simulink model "modelling"  (R2024b)
settings: Solver=VariableStepAuto  StartTime=0.0  StopTime=10.0  RelTol=1e-3
InitFcn:
  | Init
  | Observer_and_complementary_filter
undefined symbols (not defined in the file): body, C, denH, denHw, DiscIntNeverNeededParam, drv, dspblkCoreblockFVToolHelper, Fv, g, gbox, gcbh, M11, M22, mot, ms22g, numH, numHw, sens, Ts, wheel
libraries: simulink_extras x4
settings Model: Creator=UTENTE041019  LastModifiedBy=lucag

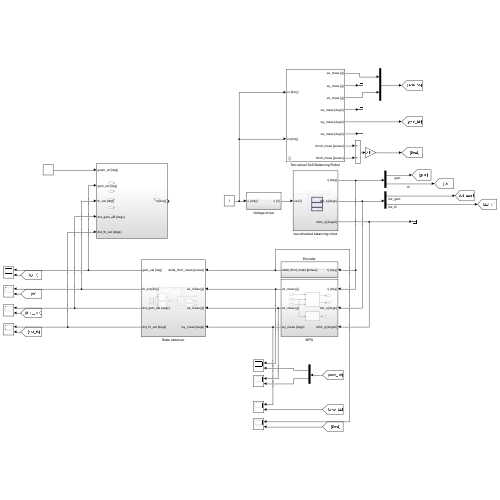
[thumbnail: Simulink's stored preview of the top-level diagram]
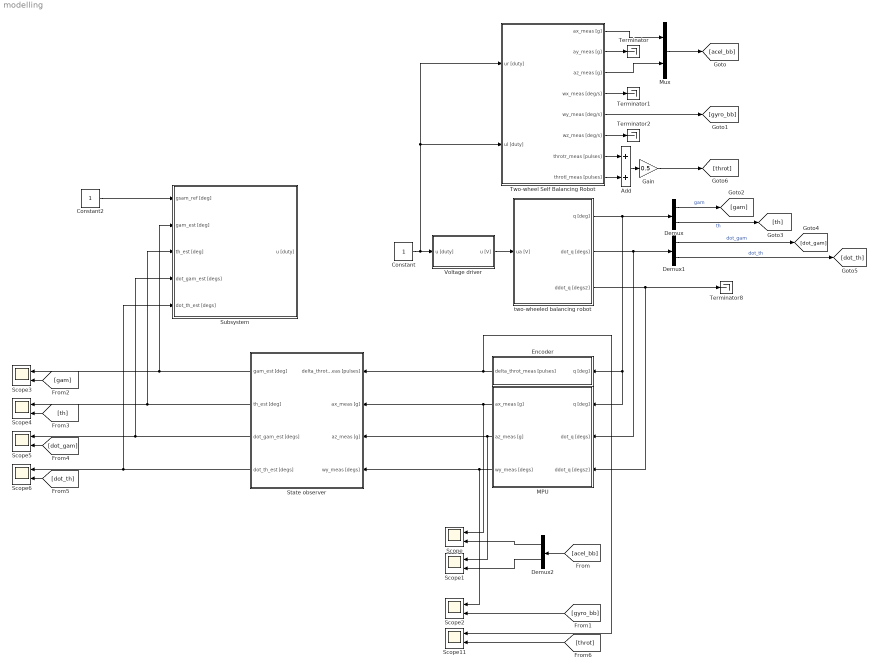
== system modelling ==
  Add : Sum
  Constant : Constant
  Constant2 : Constant
  Demux : Demux  Outputs=2
  Demux1 : Demux  Outputs=2
  Demux2 : Demux  Outputs=2
  Encoder : Subsystem
  Gain : Gain  Gain=0.5
  MPU : Subsystem
  Mux : Mux  Inputs=2
  Scope{,1..6,11} (8 alike) : Scope  NumInputPorts=2
  State observer : Subsystem
  Subsystem : Subsystem
  Terminator{,1..2,8} (4 alike) : Terminator
  "Two-wheel Self Balancing Robot " : Subsystem  mask(Balancing robot (longitudinal + lateral dynamics)){initState=[0, 0, 0, 0, 0, 0], Ts=0.01}
      mask prompts: initState "Initial state [gam(0), psi(0), th(0), dot_gam(0), dot_psi(0), dot_th(0)]'"; Ts "Sample time:"
      mask help:
      | Balancing robot dynamic model.
      | Includes both the longitudinal and lateral (yaw) dynamics.
      mask init:
      | %% General parameters and conversion gains
      | 
      | %   gravity acc [m/s^2]
      | g = 9.81;
      | 
      | %   conversion gains
      | rpm2rads = 2*pi/60;         %   [rpm]   -> [rad/s]
      | rads2rpm = 60/2/pi;         %   [rad/s] -> [rpm]
      | rpm2degs = 360/60;          %   [rpm]   -> [deg/s]
      | degs2rpm = 60/360;          %   [deg/s] -> [rpm]
      | deg2rad = pi/180;           %   [deg]   -> [rad]
      | rad2deg = 180/pi;           %   [rad]   -> [deg]
      | g2ms2 = g;                  %   [acc_g] -> [m/s^2]
      | ms22g = 1/g;                %   [m/s^2] -> [acc_g]
      | ozin2Nm = 0.706e-2;         %   [oz*inch] -> [N*m]
      | 
      | 
      | %%  Battery data
      | 
      | %   electrical data
      | batt.UN = 11.1;     %   nominal voltage
      | 
      | 
      | %%  H-bridge PWM voltage driver
      | 
      | drv.Vbus = batt.UN;                     %   H-bridge DC bus voltage  
      | drv.pwm.bits = 8;                       %   PWM resolution [bits]
      | drv.pwm.levels = 2^drv.pwm.bits;        %   PWM levels
      | drv.pwm.Fs = 490;                       %   PWM frequency
      | drv.dutymax = drv.pwm.levels-1;         %   max duty cycle code
      | drv.duty2V = drv.Vbus/drv.dutymax;      %   duty cycle code (0-255) to voltage
      | drv.V2duty = drv.dutymax/drv.Vbus;      %   voltage to duty cycle code (0-255)
      | 
      | 
      | %%  Gearbox data 
      | 
      | gbox.N = 30;            %   reduction ratio
      | 
      | 
      | %%  Sensors data - Hall-effect encoder
      | 
      | %   Hall-effect encoder
      | sens.enc.ppr = 16*4;    %   pulses per rotation at motor side (w/ quadrature decoding)
      | sens.enc.pulse2deg = 360/sens.enc.ppr;
      | sens.enc.pulse2rad = 2*pi/sens.enc.ppr;
      | sens.enc.deg2pulse = sens.enc.ppr/360;
      | sens.enc.rad2pulse = sens.enc.ppr/2/pi;
      | 
      | 
      | %%  Sensors data - MPU6050 (accelerometer + gyro)
      | 
      | %   center of mass (CoM) position
      | sens.mpu.xb = 0;
      | sens.mpu.yb = 0;
      | sens.mpu.zb = 13.5e-3;
      | 
      | %       MPU6050 embedded accelerometer specs
      | sens.mpu.acc.bits = 16;
      | sens.mpu.acc.fs_g = 16;                                                         %   full-scale in "g" units
      | sens.mpu.acc.fs = sens.mpu.acc.fs_g * g2ms2;                                    %   full-scale in [m/s^2] 
      | sens.mpu.acc.g2LSB = floor(2^(sens.mpu.acc.bits-1)/sens.mpu.acc.fs_g);          %   sensitivity [LSB/g]
      | sens.mpu.acc.ms22LSB = sens.mpu.acc.g2LSB * ms22g;                              %   sensitvity [LSB/(m/s^2)]
      | sens.mpu.acc.LSB2g = sens.mpu.acc.fs_g/2^(sens.mpu.acc.bits-1);                 %   output quantization step [g/LSB]
      | sens.mpu.acc.LSB2ms2 = sens.mpu.acc.LSB2g * g2ms2;                              %   output quantization step [ms2/LSB]
      | sens.mpu.acc.bw = 94;                                                           %   output low-pass filter bandwidth
      | sens.mpu.acc.noisestd = 400e-6*sqrt(100);                                       %   output noise std [g-rms]
      | sens.mpu.acc.noisevar = sens.mpu.acc.noisestd^2;                                %   output noise var [g^2]
      | 
      | %       MPU6050 embdedded gyroscope specs
      | sens.mpu.gyro.bits = 16;
      | sens.mpu.gyro.fs_degs = 250;                                                    %   full scale in [deg/s (dps)]
      | sens.mpu.gyro.fs = sens.mpu.gyro.fs_degs * deg2rad;                             %   full scale in [rad/s]
      | sens.mpu.gyro.degs2LSB = floor(2^(sens.mpu.gyro.bits-1)/sens.mpu.gyro.fs_degs);	%   sensitivity [LSB/degs]
      | sens.mpu.gyro.rads2LSB = sens.mpu.gyro.degs2LSB * rad2deg;                      %   sensitivity [LSB/rads] 
      | sens.mpu.gyro.LSB2degs = sens.mpu.gyro.fs_degs/2^(sens.mpu.gyro.bits-1);        %   output quantization step [degs/LSB]
      | sens.mpu.gyro.LSB2rads = sens.mpu.gyro.LSB2degs * deg2rad;                      %   output quantization step [rads/LSB]
      | sens.mpu.gyro.bw = 98;                                                          %   output low-pass filter bandwidth
      | sens.mpu.gyro.noisestd = 5e-3*sqrt(100);                                        %   output noise std [degs-rms]
      | sens.mpu.gyro.noisevar = sens.mpu.acc.noisestd ^2;                              %   output noise var [degs^2]
      mask Help:
      | Riccardo Antonello (antonello@dei.unipd.it)
      | 
      | May 19, 2020
      | 
      | Dept. of Information Engineering, University of Padova
  Voltage driver : Subsystem
  two-wheeled balancing robot : Subsystem
  wires:
  Voltage driver/1(u [V]) -> two-wheeled balancing robot/1(ua [V])
  two-wheeled balancing robot/1(q [deg]) -> MPU/1(q [deg]), Encoder/1(q [deg]), Demux/1
  two-wheeled balancing robot/2(dot_q [degs]) -> MPU/2(dot_q [degs]), Demux1/1
  two-wheeled balancing robot/3(ddot_q [degs2]) -> Terminator8/1, MPU/3(ddot_q [degs2])
  Constant/1 -> "Two-wheel Self Balancing Robot "/1(ur [duty]), "Two-wheel Self Balancing Robot "/2(ul [duty]), Voltage driver/1(u [duty])
  Demux/1 -> [gam]  "gam"
  Demux/2 -> [th]  "th"
  Demux1/2 -> [dot_th]  "dot_th"
  Demux1/1 -> [dot_gam]  "dot_gam"
  Encoder/1(delta_throt_meas [pulses]) -> Scope11/1, State observer/1(delta_throt_meas [pulses])
  MPU/1(ax_meas [g]) -> Scope/1, State observer/2(ax_meas [g])
  MPU/2(az_meas [g]) -> Scope1/1, State observer/3(az_meas [g])
  MPU/3(wy_meas [degs]) -> Scope2/1, State observer/4(wy_meas [degs])
  State observer/1(gam_est [deg]) -> Scope3/1, Subsystem/2(gam_est [deg])
  State observer/2(th_est [deg]) -> Scope4/1, Subsystem/3(th_est [deg])
  State observer/3(dot_gam_est [degs]) -> Subsystem/4(dot_gam_est [degs]), Scope5/1
  State observer/4(dot_th_est [degs]) -> Subsystem/5(dot_th_est [degs]), Scope6/1
  Constant2/1 -> Subsystem/1(gsam_ref [deg])
  [acel_bb] -> Demux2/1
  Demux2/1 -> Scope/2
  Demux2/2 -> Scope1/2
  [gyro_bb] -> Scope2/2
  [gam] -> Scope3/2
  [th] -> Scope4/2
  [dot_gam] -> Scope5/2
  [dot_th] -> Scope6/2
  "Two-wheel Self Balancing Robot "/2(ay_meas [g]) -> Terminator/1
  "Two-wheel Self Balancing Robot "/4(wx_meas [deg/s]) -> Terminator1/1
  "Two-wheel Self Balancing Robot "/6(wz_meas [deg/s]) -> Terminator2/1
  "Two-wheel Self Balancing Robot "/7(throtr_meas [pulses]) -> Add/1
  "Two-wheel Self Balancing Robot "/8(throtl_meas [pulses]) -> Add/2
  Add/1 -> Gain/1
  "Two-wheel Self Balancing Robot "/1(ax_meas [g]) -> Mux/1
  "Two-wheel Self Balancing Robot "/3(az_meas [g]) -> Mux/2
  Mux/1 -> [acel_bb]
  "Two-wheel Self Balancing Robot "/5(wy_meas [deg/s]) -> [gyro_bb]
  Gain/1 -> [throt]
  [throt] -> Scope11/2

== system modelling/Encoder ==
  q [deg] : Inport
  Gain : Gain  Gain=[1 -1]  Multiplication=Matrix(K*u)
  Gain1 : Gain  Gain=gbox.N
  Gain2 : Gain  Gain=sens.enc.deg2pulse
  Quantizer : Quantizer  QuantizationInterval=sens.enc.pulse2deg
  Zero-Order Hold : ZeroOrderHold  SampleTime=Ts
  delta_throt_meas [pulses] : Outport
  wires:
  Quantizer/1 -> Gain2/1
  Gain1/1 -> Zero-Order Hold/1
  Zero-Order Hold/1 -> Quantizer/1
  Gain/1 -> Gain1/1
  q [deg]/1 -> Gain/1
  Gain2/1 -> delta_throt_meas [pulses]/1

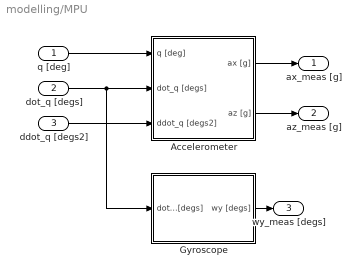
== system modelling/MPU ==
  q [deg] : Inport
  dot_q [degs] : Inport  Port=2
  ddot_q [degs2] : Inport  Port=3
  Accelerometer : Subsystem
  Gyroscope : Subsystem
  ax_meas [g] : Outport
  az_meas [g] : Outport  Port=2
  wy_meas [degs] : Outport  Port=3
  wires:
  dot_q [degs]/1 -> Gyroscope/1(dot_q [degs]), Accelerometer/2(dot_q [degs])
  ddot_q [degs2]/1 -> Accelerometer/3(ddot_q [degs2])
  Accelerometer/2(az [g]) -> az_meas [g]/1
  Accelerometer/1(ax [g]) -> ax_meas [g]/1
  Gyroscope/1(wy [degs]) -> wy_meas [degs]/1
  q [deg]/1 -> Accelerometer/1(q [deg])

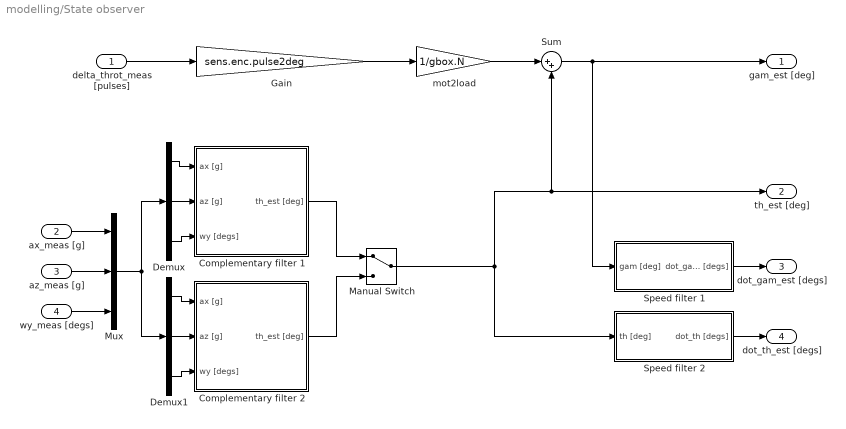
== system modelling/State observer ==
  delta_throt_meas [pulses] : Inport
  ax_meas [g] : Inport  Port=2
  az_meas [g] : Inport  Port=3
  wy_meas [degs] : Inport  Port=4
  Complementary filter 1 : Subsystem
  Complementary filter 2 : Subsystem
  Demux : Demux  Outputs=3
  Demux1 : Demux  Outputs=3
  Gain : Gain  Gain=sens.enc.pulse2deg
  Manual Switch : ManualSwitch
  Mux : Mux  Inputs=3
  Speed filter 1 : Subsystem
  Speed filter 2 : Subsystem
  Sum : Sum  Inputs=|++
  mot2load : Gain  Gain=1/gbox.N
  gam_est [deg] : Outport
  th_est [deg] : Outport  Port=2
  dot_gam_est [degs] : Outport  Port=3
  dot_th_est [degs] : Outport  Port=4
  wires:
  delta_throt_meas [pulses]/1 -> Gain/1
  Gain/1 -> mot2load/1
  mot2load/1 -> Sum/1
  Sum/1 -> Speed filter 1/1(gam [deg]), gam_est [deg]/1
  Speed filter 1/1(dot_gam [degs]) -> dot_gam_est [degs]/1
  Speed filter 2/1(dot_th [degs]) -> dot_th_est [degs]/1
  ax_meas [g]/1 -> Mux/1
  az_meas [g]/1 -> Mux/2
  wy_meas [degs]/1 -> Mux/3
  Demux/1 -> Complementary filter 1/1(ax [g])
  Demux/3 -> Complementary filter 1/3(wy [degs])
  Demux/2 -> Complementary filter 1/2(az [g])
  Demux1/2 -> Complementary filter 2/2(az [g])
  Demux1/1 -> Complementary filter 2/1(ax [g])
  Demux1/3 -> Complementary filter 2/3(wy [degs])
  Mux/1 -> Demux/1, Demux1/1
  Complementary filter 1/1(th_est [deg]) -> Manual Switch/1
  Complementary filter 2/1(th_est [deg]) -> Manual Switch/2
  Manual Switch/1 -> Sum/2, th_est [deg]/1, Speed filter 2/1(th [deg])

== system modelling/Subsystem ==
  gsam_ref [deg] : Inport
  gam_est [deg] : Inport  Port=2
  th_est [deg] : Inport  Port=3
  dot_gam_est [degs] : Inport  Port=4
  dot_th_est [degs] : Inport  Port=5
  u [duty] : Outport

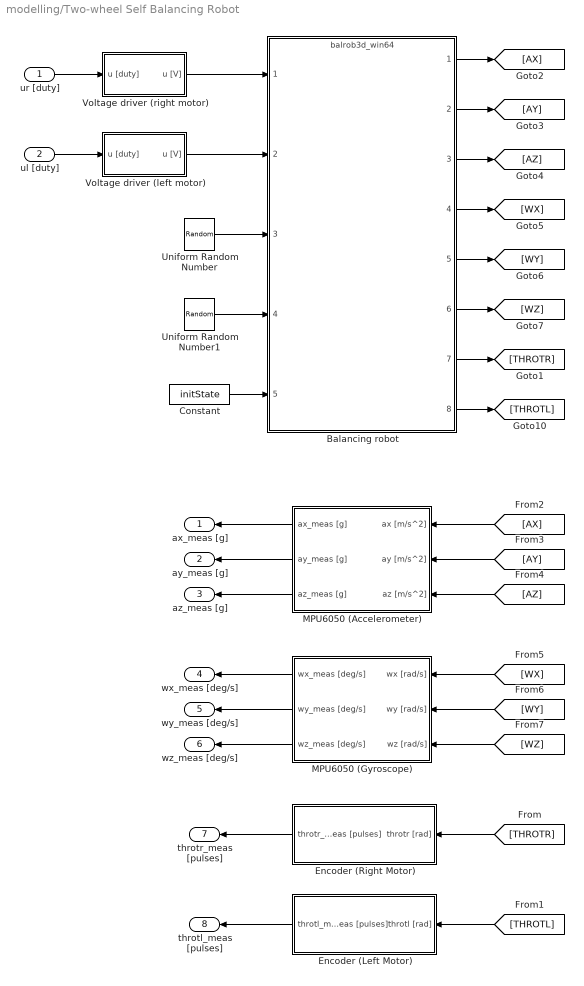
== system modelling/Two-wheel Self Balancing Robot  ==
  ur [duty] : Inport
  ul [duty] : Inport  Port=2
  Balancing robot : ModelReference  ModelNameDialog=balrob3d_win64.slxp  ModelReferenceVersion=1.741  CopyOfModelProtected=on
  Constant : Constant  Value=initState
  Encoder (Left Motor) : Subsystem
  Encoder (Right Motor) : Subsystem
  MPU6050 (Accelerometer) : Subsystem
  MPU6050 (Gyroscope) : Subsystem
  Uniform Random Number : UniformRandomNumber  Minimum=0.7  Maximum=1.3  SampleTime=1
  Uniform Random Number1 : UniformRandomNumber  Minimum=0.7  Maximum=1.3  Seed=10  SampleTime=1
  Voltage driver (left motor) : Subsystem
  Voltage driver (right motor) : Subsystem
  ax_meas [g] : Outport
  ay_meas [g] : Outport  Port=2
  az_meas [g] : Outport  Port=3
  wx_meas [deg/s] : Outport  Port=4
  wy_meas [deg/s] : Outport  Port=5
  wz_meas [deg/s] : Outport  Port=6
  throtr_meas [pulses] : Outport  Port=7
  throtl_meas [pulses] : Outport  Port=8
  wires:
  ur [duty]/1 -> Voltage driver (right motor)/1(u [duty])
  [WX] -> MPU6050 (Gyroscope)/1(wx [rad/s])
  Balancing robot/2 -> [AY]
  Balancing robot/4 -> [WX]
  Balancing robot/8 -> [THROTL]
  Balancing robot/1 -> [AX]
  [THROTL] -> Encoder (Left Motor)/1(throtl [rad])
  Balancing robot/6 -> [WZ]
  Balancing robot/7 -> [THROTR]
  Balancing robot/5 -> [WY]
  [AX] -> MPU6050 (Accelerometer)/1(ax [m/s^2])
  [WY] -> MPU6050 (Gyroscope)/2(wy [rad/s])
  Balancing robot/3 -> [AZ]
  [WZ] -> MPU6050 (Gyroscope)/3(wz [rad/s])
  [AZ] -> MPU6050 (Accelerometer)/3(az [m/s^2])
  [THROTR] -> Encoder (Right Motor)/1(throtr [rad])
  ul [duty]/1 -> Voltage driver (left motor)/1(u [duty])
  [AY] -> MPU6050 (Accelerometer)/2(ay [m/s^2])
  MPU6050 (Accelerometer)/1(ax_meas [g]) -> ax_meas [g]/1
  MPU6050 (Accelerometer)/2(ay_meas [g]) -> ay_meas [g]/1
  MPU6050 (Accelerometer)/3(az_meas [g]) -> az_meas [g]/1
  MPU6050 (Gyroscope)/1(wx_meas [deg/s]) -> wx_meas [deg/s]/1
  MPU6050 (Gyroscope)/2(wy_meas [deg/s]) -> wy_meas [deg/s]/1
  MPU6050 (Gyroscope)/3(wz_meas [deg/s]) -> wz_meas [deg/s]/1
  Encoder (Right Motor)/1(throtr_meas [pulses]) -> throtr_meas [pulses]/1
  Encoder (Left Motor)/1(throtl_meas [pulses]) -> throtl_meas [pulses]/1
  Voltage driver (right motor)/1(u [V]) -> Balancing robot/1
  Voltage driver (left motor)/1(u [V]) -> Balancing robot/2
  Uniform Random Number/1 -> Balancing robot/3
  Uniform Random Number1/1 -> Balancing robot/4
  Constant/1 -> Balancing robot/5

== system modelling/Voltage driver ==
  u [duty] : Inport
  " " : Gain  Gain=drv.duty2V
  Rounding Function : Rounding  Operator=fix
  Saturation : Saturate  UpperLimit=drv.dutymax  LowerLimit=-drv.dutymax
  Saturation1 : Saturate  UpperLimit=drv.Vbus  LowerLimit=-drv.Vbus
  Zero-Order Hold : ZeroOrderHold  SampleTime=Ts
  u [V] : Outport
  wires:
  Rounding Function/1 -> " "/1
  " "/1 -> Saturation1/1
  Saturation1/1 -> Zero-Order Hold/1
  u [duty]/1 -> Saturation/1
  Saturation/1 -> Rounding Function/1
  Zero-Order Hold/1 -> u [V]/1

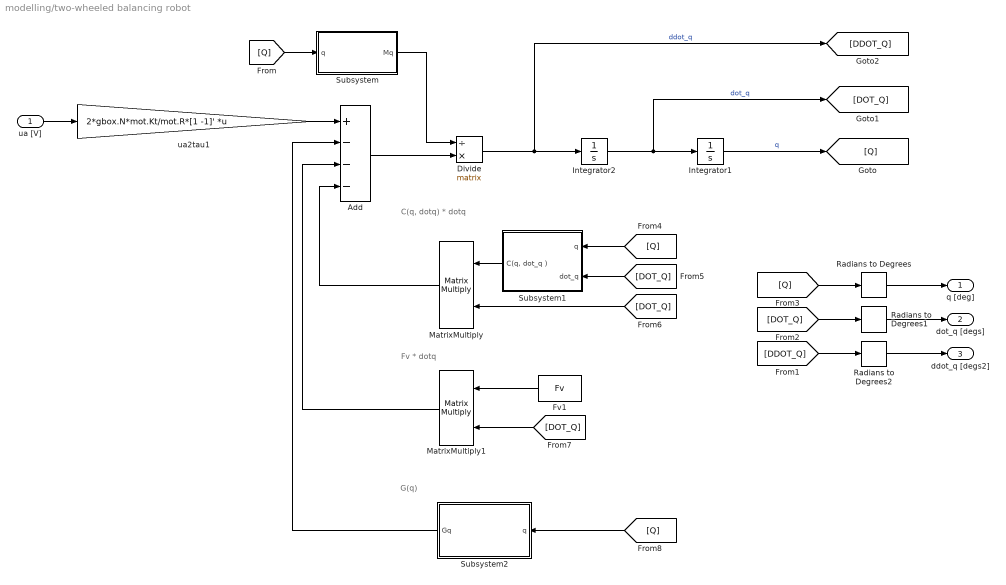
== system modelling/two-wheeled balancing robot ==
  note: G(q)
  note: Fv * dotq
  note: C(q, dotq) * dotq
  ua [V] : Inport
  Add : Sum  Inputs=+---
  Divide : Product  Inputs=/*  Multiplication=Matrix(*)
  Fv1 : Constant  Value=Fv
  Integrator1 : Integrator  InitialCondition=[0 0]'
  Integrator2 : Integrator  InitialCondition=[0 0]'
  MatrixMultiply : Product  Multiplication=Matrix(*)
  MatrixMultiply1 : Product  Multiplication=Matrix(*)
  Radians to Degrees : simulink_extras/Transformations/Radians to Degrees
  Radians to Degrees1 : simulink_extras/Transformations/Radians to Degrees
  Radians to Degrees2 : simulink_extras/Transformations/Radians to Degrees
  Subsystem : Subsystem
  Subsystem1 : Subsystem
  Subsystem2 : Subsystem
  ua2tau1 : Gain  Gain=2*gbox.N*mot.Kt/mot.R*[1 -1]'  Multiplication=Matrix(K*u)
  q [deg] : Outport
  dot_q [degs] : Outport  Port=2
  ddot_q [degs2] : Outport  Port=3
  wires:
  Subsystem1/1("C(q, dot_q )") -> MatrixMultiply/1
  Integrator2/1 -> [DOT_Q], Integrator1/1  "dot_q"
  Add/1 -> Divide/2
  [DOT_Q] -> Radians to Degrees1/1
  Divide/1 -> Integrator2/1, [DDOT_Q]  "ddot_q"
  Integrator1/1 -> [Q]  "q"
  ua2tau1/1 -> Add/1
  Radians to Degrees/1 -> q [deg]/1
  ua [V]/1 -> ua2tau1/1
  [Q] -> Subsystem1/1(q)
  Radians to Degrees1/1 -> dot_q [degs]/1
  Radians to Degrees2/1 -> ddot_q [degs2]/1
  [Q] -> Radians to Degrees/1
  [DDOT_Q] -> Radians to Degrees2/1
  MatrixMultiply/1 -> Add/4
  MatrixMultiply1/1 -> Add/3
  [DOT_Q] -> MatrixMultiply/2
  Subsystem2/1(Gq) -> Add/2
  [DOT_Q] -> MatrixMultiply1/2
  [Q] -> Subsystem/1(q)
  [DOT_Q] -> Subsystem1/2(dot_q)
  Subsystem/1(Mq) -> Divide/1
  [Q] -> Subsystem2/1(q)
  Fv1/1 -> MatrixMultiply1/1

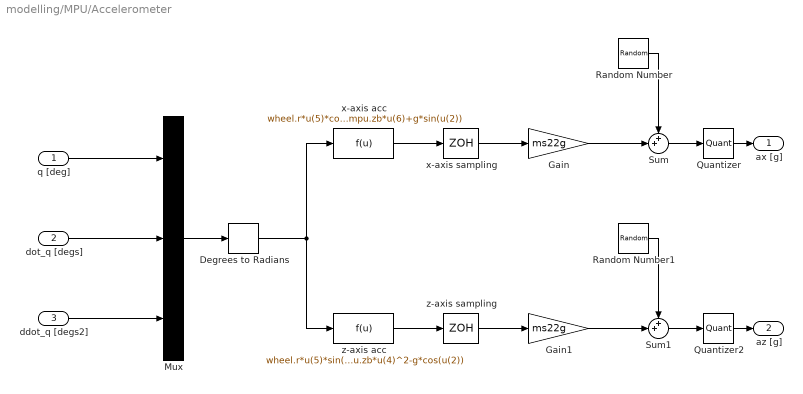
== system modelling/MPU/Accelerometer ==
  q [deg] : Inport
  dot_q [degs] : Inport  Port=2
  ddot_q [degs2] : Inport  Port=3
  Degrees to Radians : simulink_extras/Transformations/Degrees to Radians
  Gain : Gain  Gain=ms22g
  Gain1 : Gain  Gain=ms22g
  Mux : Mux  Inputs=3
  Quantizer : Quantizer  QuantizationInterval=sens.mpu.acc.LSB2g
  Quantizer2 : Quantizer  QuantizationInterval=sens.mpu.acc.LSB2g
  Random Number : RandomNumber  Variance=sens.mpu.acc.noisevar  SampleTime=Ts
  Random Number1 : RandomNumber  Variance=sens.mpu.acc.noisevar  SampleTime=Ts
  Sum : Sum  Inputs=++|
  Sum1 : Sum  Inputs=++|
  x-axis acc : Fcn  Expr=wheel.r*u(5)*cos(u(2))+sens.mpu.zb*u(6)+g*sin(u(2))
  x-axis sampling : ZeroOrderHold  SampleTime=Ts
  z-axis acc : Fcn  Expr=wheel.r*u(5)*sin(u(2))-sens.mpu.zb*u(4)^2-g*cos(u(2))
  z-axis sampling : ZeroOrderHold  SampleTime=Ts
  ax [g] : Outport
  az [g] : Outport  Port=2
  wires:
  Quantizer2/1 -> az [g]/1
  Gain/1 -> Sum/2
  Sum/1 -> Quantizer/1
  Random Number1/1 -> Sum1/1
  x-axis acc/1 -> x-axis sampling/1
  ddot_q [degs2]/1 -> Mux/3
  z-axis sampling/1 -> Gain1/1
  Sum1/1 -> Quantizer2/1
  Gain1/1 -> Sum1/2
  z-axis acc/1 -> z-axis sampling/1
  x-axis sampling/1 -> Gain/1
  Mux/1 -> Degrees to Radians/1
  dot_q [degs]/1 -> Mux/2
  Random Number/1 -> Sum/1
  Quantizer/1 -> ax [g]/1
  q [deg]/1 -> Mux/1
  Degrees to Radians/1 -> z-axis acc/1, x-axis acc/1

== system modelling/MPU/Gyroscope ==
  dot_q [degs] : Inport
  Quantizer1 : Quantizer  QuantizationInterval=sens.mpu.gyro.LSB2degs
  Random Number2 : RandomNumber  Variance=sens.mpu.gyro.noisevar  SampleTime=Ts
  Selector : Gain  Gain=[0 1]  Multiplication=Matrix(K*u)
  Sum2 : Sum  Inputs=++|
  Y-axis sampling : ZeroOrderHold  SampleTime=Ts
  wy [degs] : Outport
  wires:
  Selector/1 -> Y-axis sampling/1
  Sum2/1 -> Quantizer1/1
  Random Number2/1 -> Sum2/1
  Y-axis sampling/1 -> Sum2/2
  Quantizer1/1 -> wy [degs]/1
  dot_q [degs]/1 -> Selector/1

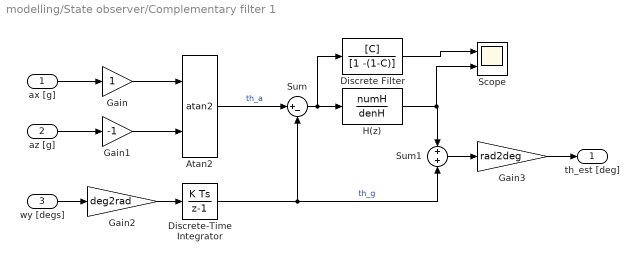
== system modelling/State observer/Complementary filter 1 ==
  ax [g] : Inport
  az [g] : Inport  Port=2
  wy [degs] : Inport  Port=3
  Atan2 : Trigonometry  Operator=atan2
  Discrete Filter : DiscreteFilter  LoadFcn=dspblkCoreblockFVToolHelper(gcbh,'load');  Numerator=[C]  Denominator=[1 -(1-C)]
      settings: CopyFcn=dspblkCoreblockFVToolHelper(gcbh,'copy');  DeleteFcn=dspblkCoreblockFVToolHelper(gcbh,'close');  ModelCloseFcn=dspblkCoreblockFVToolHelper(gcbh,'close');  PreSaveFcn=dspblkCoreblockFVToolHelper(gcbh,'presave');  PostSaveFcn=dspblkCoreblockFVToolHelper(gcbh,'postsave');  CloseFcn=dspblkCoreblockFVToolHelper(gcbh,'close');
  Discrete-Time Integrator : DiscreteIntegrator  SampleTime=Ts  ICPrevOutput=DiscIntNeverNeededParam  ICPrevScaledInput=DiscIntNeverNeededParam
  Gain : Gain
  Gain1 : Gain  Gain=-1
  Gain2 : Gain  Gain=deg2rad
  Gain3 : Gain  Gain=rad2deg
  H(z) : DiscreteTransferFcn  Numerator=numH  Denominator=denH
  Scope : Scope  NumInputPorts=2
  Sum : Sum  Inputs=|+-
  Sum1 : Sum  Inputs=+|+
  th_est [deg] : Outport
  wires:
  ax [g]/1 -> Gain/1
  az [g]/1 -> Gain1/1
  Gain/1 -> Atan2/1
  Gain1/1 -> Atan2/2
  Atan2/1 -> Sum/1  "th_a"
  wy [degs]/1 -> Gain2/1
  Gain2/1 -> Discrete-Time Integrator/1
  Discrete-Time Integrator/1 -> Sum1/2, Sum/2  "th_g"
  Sum/1 -> Discrete Filter/1, H(z)/1
  H(z)/1 -> Scope/2, Sum1/1
  Sum1/1 -> Gain3/1
  Gain3/1 -> th_est [deg]/1
  Discrete Filter/1 -> Scope/1

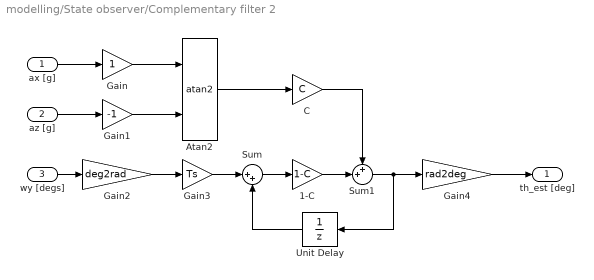
== system modelling/State observer/Complementary filter 2 ==
  ax [g] : Inport
  az [g] : Inport  Port=2
  wy [degs] : Inport  Port=3
  1-C : Gain  Gain=1-C
  Atan2 : Trigonometry  Operator=atan2
  C : Gain  Gain=C
  Gain : Gain
  Gain1 : Gain  Gain=-1
  Gain2 : Gain  Gain=deg2rad
  Gain3 : Gain  Gain=Ts
  Gain4 : Gain  Gain=rad2deg
  Sum : Sum  Inputs=|++
  Sum1 : Sum  Inputs=++|
  Unit Delay : UnitDelay  SampleTime=-1  HasFrameUpgradeWarning=on
  th_est [deg] : Outport
  wires:
  Gain/1 -> Atan2/1
  az [g]/1 -> Gain1/1
  Gain1/1 -> Atan2/2
  ax [g]/1 -> Gain/1
  Atan2/1 -> C/1
  wy [degs]/1 -> Gain2/1
  Gain2/1 -> Gain3/1
  Gain3/1 -> Sum/1
  Sum/1 -> 1-C/1
  C/1 -> Sum1/1
  1-C/1 -> Sum1/2
  Sum1/1 -> Unit Delay/1, Gain4/1
  Unit Delay/1 -> Sum/2
  Gain4/1 -> th_est [deg]/1

== system modelling/State observer/Speed filter 1 ==
  gam [deg] : Inport
  Discrete Transfer Fcn : DiscreteTransferFcn  Numerator=numHw  Denominator=denHw
  Discrete Filter : DiscreteFilter  LoadFcn=dspblkCoreblockFVToolHelper(gcbh,'load');  Numerator=[1 0 0 -1]  Denominator=[3*Ts,0,0,0]  SampleTime=Ts
      settings: CopyFcn=dspblkCoreblockFVToolHelper(gcbh,'copy');  DeleteFcn=dspblkCoreblockFVToolHelper(gcbh,'close');  ModelCloseFcn=dspblkCoreblockFVToolHelper(gcbh,'close');  PreSaveFcn=dspblkCoreblockFVToolHelper(gcbh,'presave');  PostSaveFcn=dspblkCoreblockFVToolHelper(gcbh,'postsave');  CloseFcn=dspblkCoreblockFVToolHelper(gcbh,'close');
  Scope : Scope  NumInputPorts=2
  dot_gam [degs] : Outport
  wires:
  gam [deg]/1 -> Discrete Filter/1, Discrete Transfer Fcn/1
  Discrete Transfer Fcn/1 -> Scope/1, dot_gam [degs]/1
  Discrete Filter/1 -> Scope/2

== system modelling/State observer/Speed filter 2 ==
  th [deg] : Inport
  Discrete Transfer Fcn : DiscreteTransferFcn  Numerator=numHw  Denominator=denHw
  dot_th [degs] : Outport
  wires:
  th [deg]/1 -> Discrete Transfer Fcn/1
  Discrete Transfer Fcn/1 -> dot_th [degs]/1

== system modelling/Two-wheel Self Balancing Robot /Encoder (Left Motor) ==
  throtl [rad] : Inport
  Quantizer : Quantizer  QuantizationInterval=sens.enc.pulse2rad
  Zero-Order Hold : ZeroOrderHold  SampleTime=Ts
  rad2pulse : Gain  Gain=sens.enc.rad2pulse
  throtl_meas [pulses] : Outport
  wires:
  Quantizer/1 -> rad2pulse/1
  Zero-Order Hold/1 -> Quantizer/1
  throtl [rad]/1 -> Zero-Order Hold/1
  rad2pulse/1 -> throtl_meas [pulses]/1

== system modelling/Two-wheel Self Balancing Robot /Encoder (Right Motor) ==
  throtr [rad] : Inport
  Quantizer : Quantizer  QuantizationInterval=sens.enc.pulse2rad
  Zero-Order Hold : ZeroOrderHold  SampleTime=Ts
  rad2pulse : Gain  Gain=sens.enc.rad2pulse
  throtr_meas [pulses] : Outport
  wires:
  throtr [rad]/1 -> Zero-Order Hold/1
  Zero-Order Hold/1 -> Quantizer/1
  Quantizer/1 -> rad2pulse/1
  rad2pulse/1 -> throtr_meas [pulses]/1

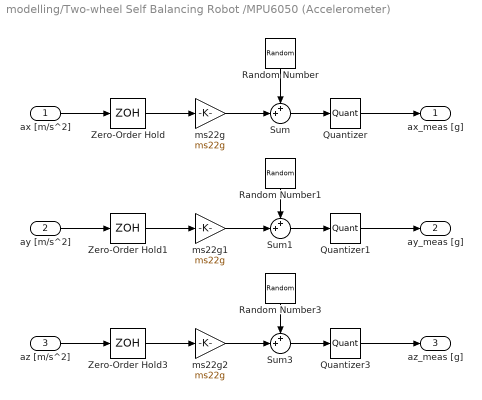
== system modelling/Two-wheel Self Balancing Robot /MPU6050 (Accelerometer) ==
  ax [m/s^2] : Inport
  ay [m/s^2] : Inport  Port=2
  az [m/s^2] : Inport  Port=3
  Quantizer : Quantizer  QuantizationInterval=sens.mpu.acc.LSB2g
  Quantizer1 : Quantizer  QuantizationInterval=sens.mpu.acc.LSB2g
  Quantizer3 : Quantizer  QuantizationInterval=sens.mpu.acc.LSB2g
  Random Number : RandomNumber  Variance=sens.mpu.acc.noisevar  Seed=1  SampleTime=Ts
  Random Number1 : RandomNumber  Variance=sens.mpu.acc.noisevar  Seed=10  SampleTime=Ts
  Random Number3 : RandomNumber  Variance=sens.mpu.acc.noisevar  Seed=100  SampleTime=Ts
  Sum : Sum  Inputs=++|
  Sum1 : Sum  Inputs=++|
  Sum3 : Sum  Inputs=++|
  Zero-Order Hold : ZeroOrderHold  SampleTime=Ts
  Zero-Order Hold1 : ZeroOrderHold  SampleTime=Ts
  Zero-Order Hold3 : ZeroOrderHold  SampleTime=Ts
  ms22g : Gain  Gain=ms22g
  ms22g1 : Gain  Gain=ms22g
  ms22g2 : Gain  Gain=ms22g
  ax_meas [g] : Outport
  ay_meas [g] : Outport  Port=2
  az_meas [g] : Outport  Port=3
  wires:
  ax [m/s^2]/1 -> Zero-Order Hold/1
  Zero-Order Hold1/1 -> ms22g1/1
  Sum1/1 -> Quantizer1/1
  ms22g/1 -> Sum/2
  ay [m/s^2]/1 -> Zero-Order Hold1/1
  Sum3/1 -> Quantizer3/1
  ms22g1/1 -> Sum1/2
  Random Number1/1 -> Sum1/1
  Random Number/1 -> Sum/1
  Sum/1 -> Quantizer/1
  Random Number3/1 -> Sum3/1
  ms22g2/1 -> Sum3/2
  Zero-Order Hold3/1 -> ms22g2/1
  az [m/s^2]/1 -> Zero-Order Hold3/1
  Zero-Order Hold/1 -> ms22g/1
  Quantizer/1 -> ax_meas [g]/1
  Quantizer1/1 -> ay_meas [g]/1
  Quantizer3/1 -> az_meas [g]/1

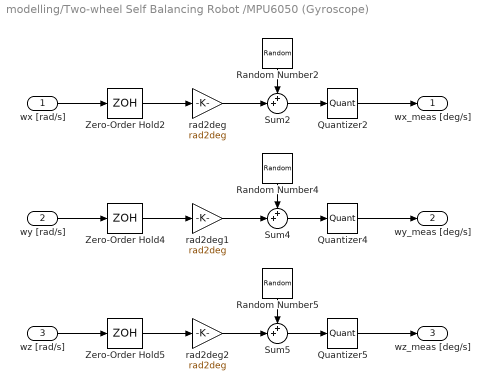
== system modelling/Two-wheel Self Balancing Robot /MPU6050 (Gyroscope) ==
  wx [rad/s] : Inport
  wy [rad/s] : Inport  Port=2
  wz [rad/s] : Inport  Port=3
  Quantizer2 : Quantizer  QuantizationInterval=sens.mpu.gyro.LSB2degs
  Quantizer4 : Quantizer  QuantizationInterval=sens.mpu.gyro.LSB2degs
  Quantizer5 : Quantizer  QuantizationInterval=sens.mpu.gyro.LSB2degs
  Random Number2 : RandomNumber  Variance=sens.mpu.gyro.noisevar  Seed=2  SampleTime=Ts
  Random Number4 : RandomNumber  Variance=sens.mpu.gyro.noisevar  Seed=20  SampleTime=Ts
  Random Number5 : RandomNumber  Variance=sens.mpu.gyro.noisevar  Seed=200  SampleTime=Ts
  Sum2 : Sum  Inputs=++|
  Sum4 : Sum  Inputs=++|
  Sum5 : Sum  Inputs=++|
  Zero-Order Hold2 : ZeroOrderHold  SampleTime=Ts
  Zero-Order Hold4 : ZeroOrderHold  SampleTime=Ts
  Zero-Order Hold5 : ZeroOrderHold  SampleTime=Ts
  rad2deg : Gain  Gain=rad2deg
  rad2deg1 : Gain  Gain=rad2deg
  rad2deg2 : Gain  Gain=rad2deg
  wx_meas [deg/s] : Outport
  wy_meas [deg/s] : Outport  Port=2
  wz_meas [deg/s] : Outport  Port=3
  wires:
  Random Number2/1 -> Sum2/1
  Sum2/1 -> Quantizer2/1
  Quantizer2/1 -> wx_meas [deg/s]/1
  Zero-Order Hold5/1 -> rad2deg2/1
  Sum4/1 -> Quantizer4/1
  rad2deg/1 -> Sum2/2
  rad2deg2/1 -> Sum5/2
  Random Number5/1 -> Sum5/1
  Zero-Order Hold4/1 -> rad2deg1/1
  Sum5/1 -> Quantizer5/1
  Random Number4/1 -> Sum4/1
  Zero-Order Hold2/1 -> rad2deg/1
  Quantizer5/1 -> wz_meas [deg/s]/1
  wz [rad/s]/1 -> Zero-Order Hold5/1
  wx [rad/s]/1 -> Zero-Order Hold2/1
  rad2deg1/1 -> Sum4/2
  Quantizer4/1 -> wy_meas [deg/s]/1
  wy [rad/s]/1 -> Zero-Order Hold4/1

== system modelling/Two-wheel Self Balancing Robot /Voltage driver (left motor) ==
  u [duty] : Inport
  Rounding Function : Rounding  Operator=fix
  Unit Delay : UnitDelay  SampleTime=1/drv.pwm.Fs  HasFrameUpgradeWarning=on
  Zero-Order Hold : ZeroOrderHold  SampleTime=Ts
  duty saturation : Saturate  UpperLimit=255  LowerLimit=-255
  duty2V : Gain  Gain=drv.duty2V
  voltage saturation : Saturate  UpperLimit=drv.Vbus  LowerLimit=-drv.Vbus
  u [V] : Outport
  wires:
  Zero-Order Hold/1 -> Unit Delay/1
  u [duty]/1 -> duty saturation/1
  voltage saturation/1 -> Zero-Order Hold/1
  duty saturation/1 -> Rounding Function/1
  Rounding Function/1 -> duty2V/1
  duty2V/1 -> voltage saturation/1
  Unit Delay/1 -> u [V]/1

== system modelling/Two-wheel Self Balancing Robot /Voltage driver (right motor) ==
  u [duty] : Inport
  Rounding Function : Rounding  Operator=fix
  Unit Delay : UnitDelay  SampleTime=1/drv.pwm.Fs  HasFrameUpgradeWarning=on
  Zero-Order Hold : ZeroOrderHold  SampleTime=Ts
  duty saturation : Saturate  UpperLimit=255  LowerLimit=-255
  duty2V : Gain  Gain=drv.duty2V
  voltage saturation : Saturate  UpperLimit=drv.Vbus  LowerLimit=-drv.Vbus
  u [V] : Outport
  wires:
  u [duty]/1 -> duty saturation/1
  duty saturation/1 -> Rounding Function/1
  Zero-Order Hold/1 -> Unit Delay/1
  voltage saturation/1 -> Zero-Order Hold/1
  Rounding Function/1 -> duty2V/1
  duty2V/1 -> voltage saturation/1
  Unit Delay/1 -> u [V]/1

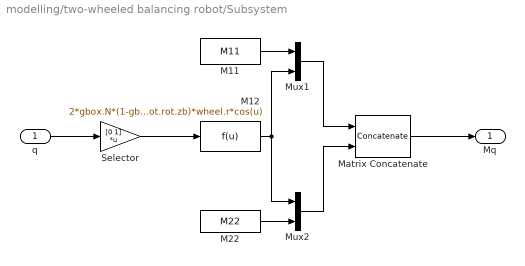
== system modelling/two-wheeled balancing robot/Subsystem ==
  q : Inport
  M11 : Constant  Value=M11
  M12 : Fcn  Expr=2*gbox.N*(1-gbox.N)*mot.rot.Iyy+(body.m*body.zb+2*mot.rot.m*mot.rot.zb)*wheel.r*cos(u)
  M22 : Constant  Value=M22
  Matrix Concatenate : Concatenate  Mode=Multidimensional array  ConcatenateDimension=2
  Mux1 : Mux  Inputs=2
  Mux2 : Mux  Inputs=2
  Selector : Gain  Gain=[0 1]  Multiplication=Matrix(K*u)
  Mq : Outport
  wires:
  Matrix Concatenate/1 -> Mq/1
  Selector/1 -> M12/1
  Mux1/1 -> Matrix Concatenate/1
  Mux2/1 -> Matrix Concatenate/2
  M12/1 -> Mux1/2, Mux2/1
  M11/1 -> Mux1/1
  M22/1 -> Mux2/2
  q/1 -> Selector/1

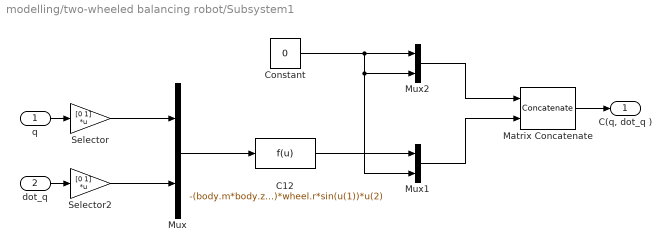
== system modelling/two-wheeled balancing robot/Subsystem1 ==
  q : Inport
  dot_q : Inport  Port=2
  C12 : Fcn  Expr=-(body.m*body.zb+2*mot.rot.m*mot.rot.zb)*wheel.r*sin(u(1))*u(2)
  Constant : Constant  Value=0
  Matrix Concatenate : Concatenate  Mode=Multidimensional array  ConcatenateDimension=2
  Mux : Mux  Inputs=2
  Mux1 : Mux  Inputs=2
  Mux2 : Mux  Inputs=2
  Selector : Gain  Gain=[0 1]  Multiplication=Matrix(K*u)
  Selector2 : Gain  Gain=[0 1]  Multiplication=Matrix(K*u)
  "C(q, dot_q )" : Outport
  wires:
  Selector2/1 -> Mux/2
  Selector/1 -> Mux/1
  Mux2/1 -> Matrix Concatenate/1
  C12/1 -> Mux1/1
  Mux/1 -> C12/1
  Constant/1 -> Mux1/2, Mux2/2, Mux2/1
  Mux1/1 -> Matrix Concatenate/2
  Matrix Concatenate/1 -> "C(q, dot_q )"/1
  q/1 -> Selector/1
  dot_q/1 -> Selector2/1

== system modelling/two-wheeled balancing robot/Subsystem2 ==
  q : Inport
  Constant : Constant  Value=0
  Gq2 : Fcn  Expr=-(body.m*body.zb+2*mot.rot.m*mot.rot.zb)*g*sin(u)
  Mux : Mux  Inputs=2
  Selector : Gain  Gain=[0 1]  Multiplication=Matrix(K*u)
  Gq : Outport
  wires:
  Constant/1 -> Mux/1
  Gq2/1 -> Mux/2
  Mux/1 -> Gq/1
  Selector/1 -> Gq2/1
  q/1 -> Selector/1
